simulink model "PIDTrajectory"  (R2022a)
settings: Solver=FixedStepAuto  StartTime=0.0  StopTime=10.0  FixedStep=1/200  RelTol=1e-3
model workspace (MAT data in the model file):
  Fa = 200
  Kd = 600
  Kp = 90000
  M = [0 0 0 0 0 0 0 0 0 0 0 0 ... (3145728 elements, 1024x1024x3)]
  TOSEND : Simulink.NumericType (value not decoded)
  axp = [0 463.62624 872.93952 1230.15168 1537.47456 1797.12 2011.29984 2182.22592 2312.11008 2403.16416 2457.6 2477.62944 ... (510 elements, 1x510)]
  ayp = [0 -0.589653333333 -1.08202666667 -1.48224 -1.79541333333 -2.02666666667 -2.18112 -2.26389333333 -2.28010666667 -2.23488 -2.13333333333 -1.98058666667 ... (510 elements, 1x510)]
  mass = 20
  server : tcpserver.internal.TCPServer (value not decoded)
  step = 0.01
  v0x = 0
  v0y = 0
  vxp = [0 2.3643136 9.0914816 19.6494336 33.5282176 50.24 69.3190656 90.3218176 112.8267776 136.4345856 160.768 185.4718976 ... (510 elements, 1x510)]
  vyp = [0 -0.00303146666667 -0.0114688 -0.0243648 -0.0408234666667 -0.06 -0.0811008 -0.103383466667 -0.1261568 -0.1487808 -0.170666666667 -0.1912768 ... (510 elements, 1x510)]
  x0 = 896
  xp = [896; 128]
  y0 = 895.999989756
  yp = [895.999989756; 128.007958323]
libraries: dspsrcs4 x6
(part 2 of 2)

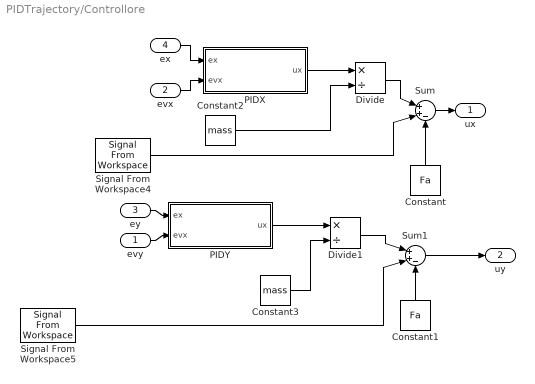
== system PIDTrajectory/Controllore ==
  evy : Inport
  evx : Inport  Port=2
  ey : Inport  Port=3
  ex : Inport  Port=4
  Constant : Constant  Value=Fa
  Constant1 : Constant  Value=Fa
  Constant2 : Constant  Value=mass
  Constant3 : Constant  Value=mass
  Divide : Product  Inputs=*/
  Divide1 : Product  Inputs=*/
  PIDX : Subsystem
  PIDY : Subsystem
  Signal From Workspace4 : dspsrcs4/Signal From Workspace  X=axp  Ts=step  nsamps=1  OutputAfterFinalValue=Setting to zero  ignoreOrWarnInputAndFrameLengths=off  OutputFrames=off
  Signal From Workspace5 : dspsrcs4/Signal From Workspace  X=ayp  Ts=step  nsamps=1  OutputAfterFinalValue=Setting to zero  ignoreOrWarnInputAndFrameLengths=off  OutputFrames=off
  Sum : Sum  Inputs=|++-
  Sum1 : Sum  Inputs=|++-
  ux : Outport
  uy : Outport  Port=2
  wires:
  ex/1 -> PIDX/1(ex)
  evx/1 -> PIDX/2(evx)
  PIDX/1(ux) -> Divide/1
  ey/1 -> PIDY/1(ex)
  evy/1 -> PIDY/2(evx)
  PIDY/1(ux) -> Divide1/1
  Sum/1 -> ux/1
  Sum1/1 -> uy/1
  Signal From Workspace5/1 -> Sum1/2
  Signal From Workspace4/1 -> Sum/2
  Constant/1 -> Sum/3
  Constant1/1 -> Sum1/3
  Divide/1 -> Sum/1
  Divide1/1 -> Sum1/1
  Constant3/1 -> Divide1/2
  Constant2/1 -> Divide/2

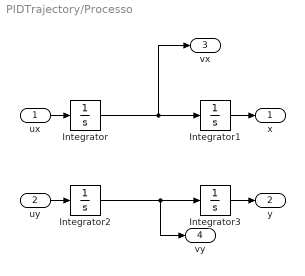
== system PIDTrajectory/Processo ==
  ux : Inport
  uy : Inport  Port=2
  Integrator : Integrator  InitialCondition=v0x
  Integrator1 : Integrator  InitialCondition=x0
  Integrator2 : Integrator  InitialCondition=v0y  UpperSaturationLimit=10  LowerSaturationLimit=-10
  Integrator3 : Integrator  InitialCondition=y0
  x : Outport  PortDimensions=1
  y : Outport  Port=2  PortDimensions=1
  vx : Outport  Port=3
  vy : Outport  Port=4
  wires:
  ux/1 -> Integrator/1
  uy/1 -> Integrator2/1
  Integrator/1 -> vx/1, Integrator1/1
  Integrator2/1 -> vy/1, Integrator3/1
  Integrator1/1 -> x/1
  Integrator3/1 -> y/1

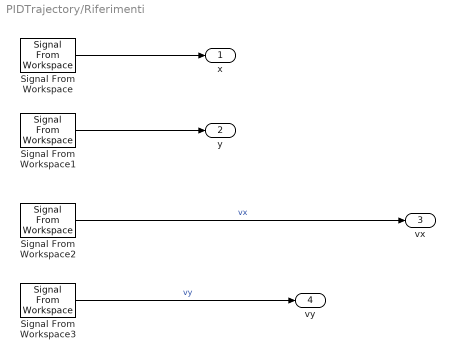
== system PIDTrajectory/Riferimenti ==
  Signal From Workspace : dspsrcs4/Signal From Workspace  X=xp  Ts=step  nsamps=1  OutputAfterFinalValue=Holding final value  ignoreOrWarnInputAndFrameLengths=off  OutputFrames=off
  Signal From Workspace1 : dspsrcs4/Signal From Workspace  X=yp  Ts=step  nsamps=1  OutputAfterFinalValue=Holding final value  ignoreOrWarnInputAndFrameLengths=off  OutputFrames=off
  Signal From Workspace2 : dspsrcs4/Signal From Workspace  X=vxp  Ts=step  nsamps=1  OutputAfterFinalValue=Setting to zero  ignoreOrWarnInputAndFrameLengths=off  OutputFrames=off
  Signal From Workspace3 : dspsrcs4/Signal From Workspace  X=vyp  Ts=step  nsamps=1  OutputAfterFinalValue=Setting to zero  ignoreOrWarnInputAndFrameLengths=off  OutputFrames=off
  x : Outport
  y : Outport  Port=2
  vx : Outport  Port=3
  vy : Outport  Port=4
  wires:
  Signal From Workspace3/1 -> vy/1  "vy"
  Signal From Workspace/1 -> x/1
  Signal From Workspace1/1 -> y/1
  Signal From Workspace2/1 -> vx/1  "vx"

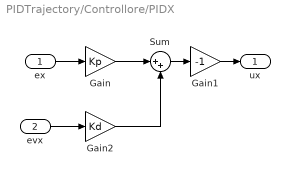
== system PIDTrajectory/Controllore/PIDX ==
  ex : Inport
  evx : Inport  Port=2
  Gain : Gain  Gain=Kp
  Gain1 : Gain  Gain=-1
  Gain2 : Gain  Gain=Kd
  Sum : Sum  Inputs=|++
  ux : Outport
  wires:
  ex/1 -> Gain/1
  Gain/1 -> Sum/1
  evx/1 -> Gain2/1
  Sum/1 -> Gain1/1
  Gain1/1 -> ux/1
  Gain2/1 -> Sum/2

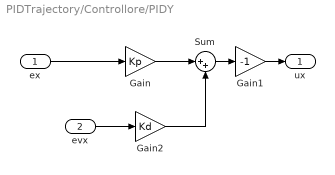
== system PIDTrajectory/Controllore/PIDY ==
  ex : Inport
  evx : Inport  Port=2
  Gain : Gain  Gain=Kp
  Gain1 : Gain  Gain=-1
  Gain2 : Gain  Gain=Kd
  Sum : Sum  Inputs=|++
  ux : Outport
  wires:
  ex/1 -> Gain/1
  Gain/1 -> Sum/1
  evx/1 -> Gain2/1
  Sum/1 -> Gain1/1
  Gain1/1 -> ux/1
  Gain2/1 -> Sum/2
